simulink model "CRUISE_WALK"  (R2024b)
settings: configuration reference "MODEL_CONFIG_CHILD" (kept outside this file)
undefined symbols (not defined in the file): MILLI_SEC_COUNTS_300_U16, SAMPLE_TIME_1MS, THROTTLE_THRESHOLD_U16, ZERO_U16
libraries: MCU_MAIN_LIB x7, simulink x6, mcbcontrolslib x4
settings Model: DataDictionary=MCU_FOC_MAIN_DD.sldd  EnableAccessToBaseWorkspace=off  Creator=415  LastModifiedBy=admin
settings ConfigSetRef: SourceName=MODEL_CONFIG_CHILD

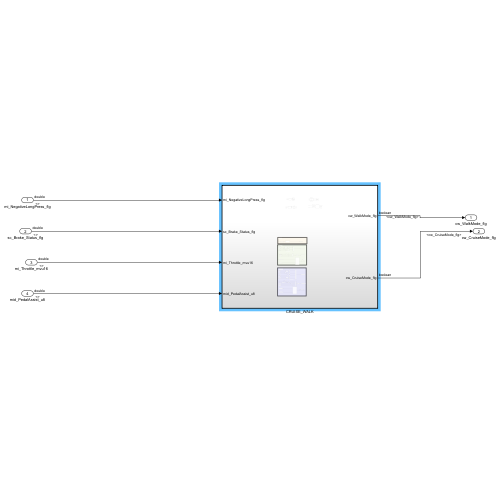
[thumbnail: Simulink's stored preview of the top-level diagram]
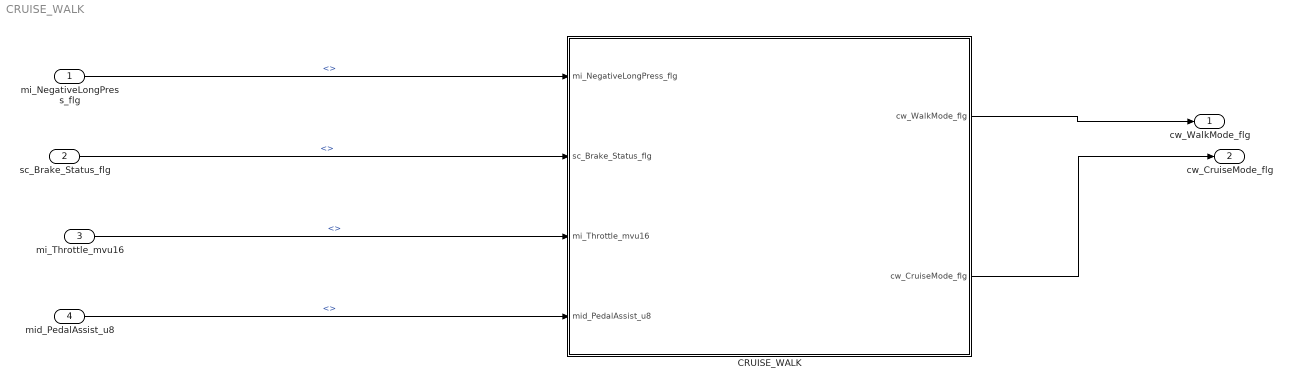
== system CRUISE_WALK ==
  mi_NegativeLongPress_flg : Inport
  sc_Brake_Status_flg : Inport  Port=2
  mi_Throttle_mvu16 : Inport  Port=3
  mid_PedalAssist_u8 : Inport  Port=4
  CRUISE_WALK : Subsystem  TreatAsAtomicUnit=on
  cw_WalkMode_flg : Outport
  cw_CruiseMode_flg : Outport  Port=2
  wires:
  CRUISE_WALK/2(cw_CruiseMode_flg) -> cw_CruiseMode_flg/1
  mid_PedalAssist_u8/1 -> CRUISE_WALK/4(mid_PedalAssist_u8)  "<>"
  mi_Throttle_mvu16/1 -> CRUISE_WALK/3(mi_Throttle_mvu16)  "<>"
  sc_Brake_Status_flg/1 -> CRUISE_WALK/2(sc_Brake_Status_flg)  "<>"
  mi_NegativeLongPress_flg/1 -> CRUISE_WALK/1(mi_NegativeLongPress_flg)  "<>"
  CRUISE_WALK/1(cw_WalkMode_flg) -> cw_WalkMode_flg/1

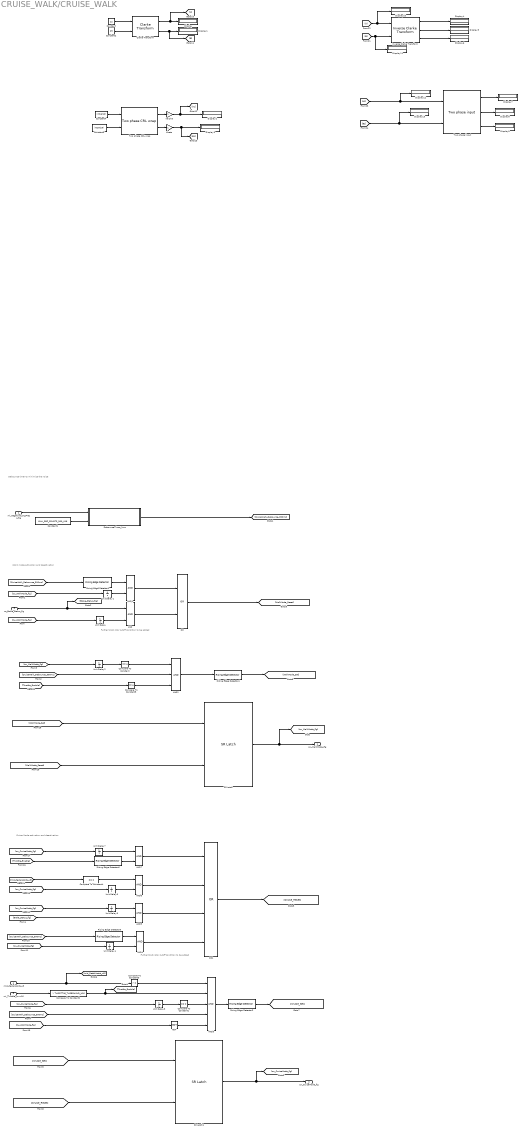
== system CRUISE_WALK/CRUISE_WALK ==
  note: Debounce timer to minimize the noise
  note: Cruise Mode activation and deactivation.
  note: Walik mode activation and deactivation
  note: Further block rotor cutoff condition to be added
  note: Further block rotor cutoff condition to be added
  mi_NegativeLongPress_flg : Inport
  sc_Brake_Status_flg : Inport  Port=2
  mi_Throttle_mvu16 : Inport  Port=3
  mid_PedalAssist_u8 : Inport  Port=4
  AND{,1,4..7} (6 alike) : Logic  AllPortsSameDT=off  OutDataTypeStr=boolean
  AND2 : Logic  Inputs=3  AllPortsSameDT=off  OutDataTypeStr=boolean
  AND3 : Logic  Inputs=5  AllPortsSameDT=off  OutDataTypeStr=boolean
  Clarke Transform : mcbcontrolslib/Clarke Transform  VariantControl=Variant2  PhaseInput=Two inputs  EnPowerInv=off
      settings: LibrarySourceBlock=mcbhdllib/Controls/Math Transforms/Clarke Transform
  Compare To Constant{,1,4..5} (4 alike) : simulink/Logic and Bit Operations/Compare To Constant  relop===  const=0  OutDataTypeStr=boolean
  Compare To Constant2 : simulink/Logic and Bit Operations/Compare To Constant  relop=>  const=THROTTLE_THRESHOLD_U16  OutDataTypeStr=boolean
  Compare To Constant3 : simulink/Logic and Bit Operations/Compare To Constant  relop=>  const=0  OutDataTypeStr=boolean
  Constant : Constant  Value=12
  Constant1 : Constant  Value=MILLI_SEC_COUNTS_300_U16
  Constant2 : Constant  Value=29
  Constant3 : Constant  Value=int16(29)
  Constant4 : Constant  Value=int16(12)
  DebounceTimer_1ms : Subsystem
  Display{,1..13} (14 alike) : Display
  From22 : From
  Goto10 : Goto
  Inverse Clarke Transform : mcbcontrolslib/Inverse Clarke Transform  PhaseInput=Two inputs  EnPowerInv=off
      settings: LibrarySourceBlock=mcbhdllib/Controls/Math Transforms/Inverse Clarke Transform
  Kalpha : Gain  RndMeth=Simplest  OutDataTypeStr=Inherit: Same as input
  Kbeta : Gain  RndMeth=Simplest  OutDataTypeStr=Inherit: Same as input
  NOT : Logic  Operator=NOT  IconShape=distinctive  AllPortsSameDT=off  OutDataTypeStr=boolean
  OR : Logic  Operator=OR  AllPortsSameDT=off  OutDataTypeStr=boolean
  OR1 : Logic  Operator=OR  Inputs=4  AllPortsSameDT=off  OutDataTypeStr=boolean
  Rising Edge Detector{1..2,4..6} (5 alike) : MCU_MAIN_LIB/Rising Edge Detector  SystemSampleTime=-1  VariantActivationTime=update diagram  AllowFlexibleInterface=on  Latency=0  AutoFrameSizeCalculation=off
  SR Latch : MCU_MAIN_LIB/SR Latch  SystemSampleTime=-1  VariantActivationTime=update diagram  AllowFlexibleInterface=on  Latency=0  AutoFrameSizeCalculation=off
  SR Latch1 : MCU_MAIN_LIB/SR Latch  SystemSampleTime=-1  VariantActivationTime=update diagram  AllowFlexibleInterface=on  Latency=0  AutoFrameSizeCalculation=off
  Two phase CRL wrap : mcbcontrolslib/Clarke Transform/Two phase input/Two phase CRL wrap  SystemSampleTime=-1  VariantActivationTime=update diagram  AllowFlexibleInterface=on  Latency=0  AutoFrameSizeCalculation=off
  Two phase input : mcbcontrolslib/Inverse Clarke Transform/Two phase input  SystemSampleTime=-1  VariantControl=Two inputs  VariantActivationTime=update diagram  AllowFlexibleInterface=on  Latency=0  AutoFrameSizeCalculation=off
  Unit Delay{,1..7} (8 alike) : UnitDelay  SampleTime=-1  HasFrameUpgradeWarning=on
  cw_WalkMode_flg : Outport
  cw_CruiseMode_flg : Outport  Port=2
  wires:
  mi_NegativeLongPress_flg/1 -> DebounceTimer_1ms/1(Enable)
  Constant1/1 -> DebounceTimer_1ms/2(SetDebounce)
  SR Latch/1 -> [cw_WalkMode_flg], cw_WalkMode_flg/1  "cw_WalkMode_flg"
  AND/1 -> OR/2  "Walk_ResetByBrake"
  [cw_WalkMode_flg] -> Unit Delay/1
  Unit Delay/1 -> AND/2
  sc_Brake_Status_flg/1 -> [Brake_Status_flg], AND/1
  Unit Delay1/1 -> AND1/2
  [cw_WalkMode_flg] -> Unit Delay1/1
  AND1/1 -> OR/1  "Walk_ResetByButton"
  Rising Edge Detector1/1 -> AND1/1
  [CruiseWalk_Debounce_300ms] -> Rising Edge Detector1/1
  DebounceTimer_1ms/1(Op) -> [CruiseWalk_Debounce_300ms]  "CruiseWalk_Debounce_300ms"
  [cw_WalkMode_flg] -> Unit Delay2/1
  Unit Delay2/1 -> Compare To Constant/1
  Compare To Constant/1 -> AND2/1
  SR Latch1/1 -> [cw_CruiseMode_flg], cw_CruiseMode_flg/1  "cw_CruiseMode_flg"
  Unit Delay3/1 -> Compare To Constant1/1
  [cw_CruiseMode_flg] -> Unit Delay3/1
  mi_Throttle_mvu16/1 -> Compare To Constant2/1
  Compare To Constant1/1 -> AND3/3
  Compare To Constant2/1 -> [Throttle_Enable], AND3/2  "Throttle_Enable"
  Compare To Constant3/1 -> AND3/1
  mid_PedalAssist_u8/1 -> [mid_PedalAssist_u8], Compare To Constant3/1
  [CruiseWalk_Debounce_300ms] -> AND2/2
  [CruiseWalk_Debounce_300ms] -> AND3/4
  [CruiseWalk_Debounce_300ms] -> Rising Edge Detector5/1
  Rising Edge Detector5/1 -> AND4/1
  [cw_CruiseMode_flg] -> Unit Delay4/1
  Unit Delay4/1 -> AND4/2
  Unit Delay5/1 -> AND5/1
  [cw_CruiseMode_flg] -> Unit Delay5/1
  Unit Delay6/1 -> AND6/2
  [cw_CruiseMode_flg] -> Unit Delay6/1
  [mid_PedalAssist_u8] -> Compare To Constant4/1
  Compare To Constant4/1 -> AND6/1
  [cw_WalkMode_flg] -> NOT/1
  NOT/1 -> AND3/5
  Rising Edge Detector6/1 -> AND7/2
  [Throttle_Enable] -> Rising Edge Detector6/1
  [cw_CruiseMode_flg] -> Unit Delay7/1
  Unit Delay7/1 -> AND7/1
  AND4/1 -> OR1/4  "Cruise_ResetByButton"
  [Brake_Status_flg] -> AND5/2
  AND7/1 -> OR1/1  "Cruise_ResetByThrottle"
  AND6/1 -> OR1/2  "Cruise_ResetByPAS"
  AND5/1 -> OR1/3  "Cruise_ResetByBrake"
  OR1/1 -> [Cruise_Reset]  "Cruise_Reset"
  [Cruise_Reset] -> SR Latch1/2
  AND3/1 -> Rising Edge Detector2/1  "Cruise_Set"
  [Cruise_Set] -> SR Latch1/1
  AND2/1 -> Rising Edge Detector4/1  "WalkMode_Set"
  [WalkMode_Set] -> SR Latch/1
  OR/1 -> [WalkMode_Reset]  "WalkMode_Reset"
  [WalkMode_Reset] -> SR Latch/2
  Rising Edge Detector2/1 -> [Cruise_Set]
  Rising Edge Detector4/1 -> [WalkMode_Set]
  Compare To Constant5/1 -> AND2/3
  [Throttle_Enable] -> Compare To Constant5/1
  Constant/1 -> Clarke Transform/1
  Constant2/1 -> Clarke Transform/2
  Clarke Transform/1 -> Goto10/1, Display/1
  Clarke Transform/2 -> [B], Display1/1
  Constant4/1 -> Two phase CRL wrap/1
  Kalpha/1 -> [A1], Display2/1
  Kbeta/1 -> Display3/1, [B1]
  Two phase CRL wrap/1 -> Kalpha/1
  Constant3/1 -> Two phase CRL wrap/2
  Two phase CRL wrap/2 -> Kbeta/1
  [A1] -> Two phase input/1, Display12/1
  [B1] -> Two phase input/2, Display13/1
  [B] -> Display11/1, Inverse Clarke Transform/2
  From22/1 -> Display10/1, Inverse Clarke Transform/1
  Inverse Clarke Transform/1 -> Display4/1
  Inverse Clarke Transform/2 -> Display5/1
  Inverse Clarke Transform/3 -> Display6/1
  Two phase input/1 -> Display7/1
  Two phase input/2 -> Display8/1
  Two phase input/3 -> Display9/1

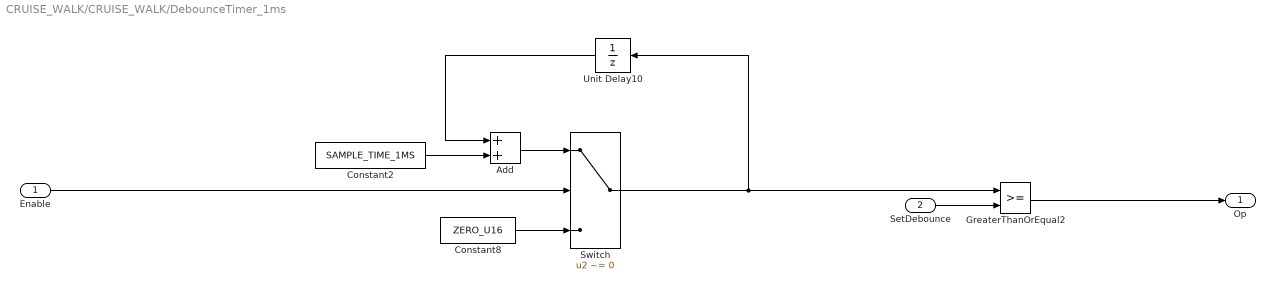
== system CRUISE_WALK/CRUISE_WALK/DebounceTimer_1ms ==
  Enable : Inport
  SetDebounce : Inport  Port=2
  Add : Sum
  Constant2 : Constant  Value=SAMPLE_TIME_1MS
  Constant8 : Constant  Value=ZERO_U16
  GreaterThanOrEqual2 : RelationalOperator  OutDataTypeStr=boolean  RndMeth=Simplest  InputSameDT=off
  Switch : Switch  Criteria=u2 ~= 0  SaturateOnIntegerOverflow=off  InputSameDT=off
  Unit Delay10 : UnitDelay  SampleTime=-1  HasFrameUpgradeWarning=on
  Op : Outport
  wires:
  Constant2/1 -> Add/2
  Enable/1 -> Switch/2
  GreaterThanOrEqual2/1 -> Op/1
  SetDebounce/1 -> GreaterThanOrEqual2/2
  Constant8/1 -> Switch/3
  Unit Delay10/1 -> Add/1
  Switch/1 -> Unit Delay10/1, GreaterThanOrEqual2/1
  Add/1 -> Switch/1
